simulink model "node"  (R2018a)
settings: Solver=VariableStepAuto  StartTime=0.0  StopTime=12000  RelTol=1e-3
libraries: dspswit3 x1
settings Model: Creator=janish  LastModifiedBy=janish

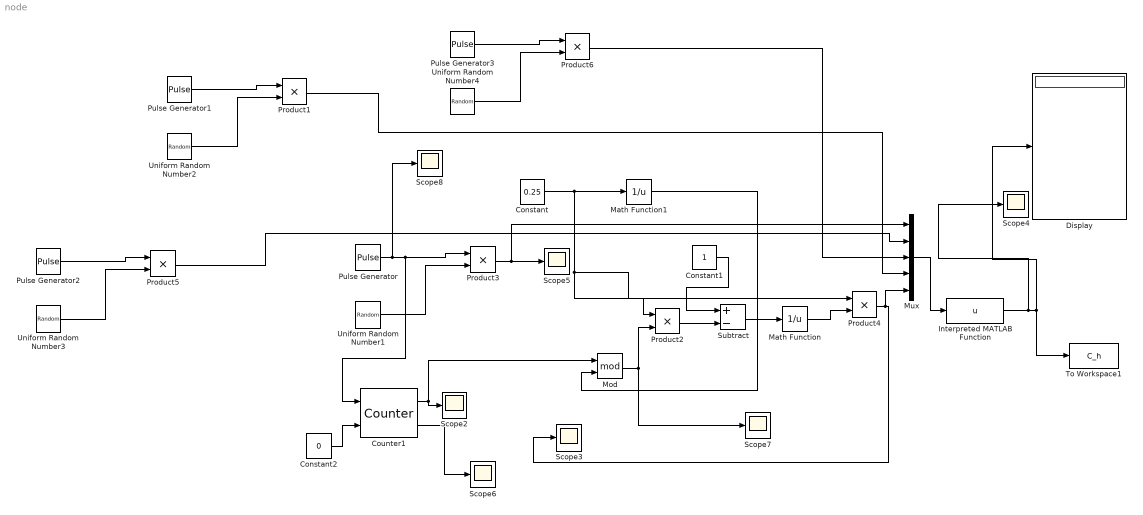
== system node ==
  Constant : Constant  Value=0.25
  Constant1 : Constant
  Constant2 : Constant  Value=0
  Counter1 : dspswit3/Counter  Direction=Up  CountEvent=Rising edge  CounterSize=32 bits  MaxCount=255  InitialCount=0  Output=Count and Hit  HitValue=32  ResetInput=on  SamplesPerFrame=1  Ts=1  CntDtype=double  HitDtype=Logical
  Display : Display
  Interpreted MATLAB Function : MATLABFcn  MATLABFcn=u
  Math Function : Math  Operator=reciprocal  RndMeth=Zero  SaturateOnIntegerOverflow=on
  Math Function1 : Math  Operator=reciprocal  RndMeth=Zero  SaturateOnIntegerOverflow=on
  Mod : Math  Operator=mod  SaturateOnIntegerOverflow=on
  Mux : Mux  Inputs=5
  Product{1..6} (6 alike) : Product
  Pulse Generator{,1..3} (4 alike) : DiscretePulseGenerator  PulseType=Time based  Period=60  PulseWidth=0.1  SampleTime=60
  Scope{2..8} (7 alike) : Scope
  Subtract : Sum  Inputs=+-
  To Workspace1 : ToWorkspace  VariableName=C_h  SampleTime=1
  Uniform Random Number1 : UniformRandomNumber  Minimum=0  SampleTime=60
  Uniform Random Number2 : UniformRandomNumber  Minimum=0  Seed=10  SampleTime=60
  Uniform Random Number3 : UniformRandomNumber  Minimum=0  Seed=20  SampleTime=60
  Uniform Random Number4 : UniformRandomNumber  Minimum=0  Seed=30  SampleTime=60
  wires:
  Product2/1 -> Subtract/2
  Product4/1 -> Mux/5, Scope3/1
  Counter1/1 -> Mod/1, Scope2/1
  Pulse Generator/1 -> Scope8/1, Counter1/1, Product3/1
  Mux/1 -> Interpreted MATLAB Function/1
  Subtract/1 -> Math Function/1
  Mod/1 -> Scope7/1, Product2/2
  Math Function1/1 -> Mod/2
  Math Function/1 -> Product4/2
  Constant1/1 -> Subtract/1
  Constant2/1 -> Counter1/2
  Uniform Random Number1/1 -> Product3/2
  Interpreted MATLAB Function/1 -> Scope4/1, To Workspace1/1, Display/1
  Constant/1 -> Product4/1, Product2/1, Math Function1/1
  Product3/1 -> Mux/1, Scope5/1
  Counter1/2 -> Scope6/1
  Pulse Generator1/1 -> Product1/1
  Uniform Random Number2/1 -> Product1/2
  Uniform Random Number3/1 -> Product5/2
  Pulse Generator2/1 -> Product5/1
  Uniform Random Number4/1 -> Product6/2
  Pulse Generator3/1 -> Product6/1
  Product6/1 -> Mux/3
  Product1/1 -> Mux/4
  Product5/1 -> Mux/2
